simulink model "IEEE_IAS_H7_LoadCurrentRefVariation"  (Simulink 9.1)
settings: Solver=VariableStepAuto  StartTime=0.0  StopTime=0.2  RelTol=1e-3
libraries: powerlib x36, powerlib_extras x3, powerlib_meascontrol x3
settings Model: Creator=mohua  LastModifiedBy=mohua
settings DataIOCC: SaveFormat=Dataset
settings OptimizationCC: LifeSpan=auto
settings DebuggingCC: UnderspecifiedInitializationDetection=Simplified  MergeDetectMultiDrivingBlocksExec=error  SFUnexpectedBacktrackingDiag=error  SFNoUnconditionalDefaultTransitionDiag=error  SFExecutionAtInitializationDiag=warning
settings HardwareCC: ProdBitPerPointer=64  ProdBitPerSizeT=64  ProdBitPerPtrDiffT=64  ProdLargestAtomicFloat=Float  ProdIntDivRoundTo=Zero  ProdEndianess=LittleEndian  ProdWordSize=64  ProdHWDeviceType=Intel->x86-64 (Windows64)
settings ModelReferenceCC: PropagateSignalLabelsOutOfModel=on
settings CodeAppCC: StateflowObjectComments=off
settings GRTTargetCC: TargetLangStandard=C99 (ISO)  CombineOutputUpdateFcns=on  GRTInterface=off
settings ConfigComp: CovMetricSettings=dwe  CovHtmlReporting=off  CovSaveCumulativeToWorkspaceVar=off  CovSaveSingleToWorkspaceVar=off  CovExternalEMLEnable=on

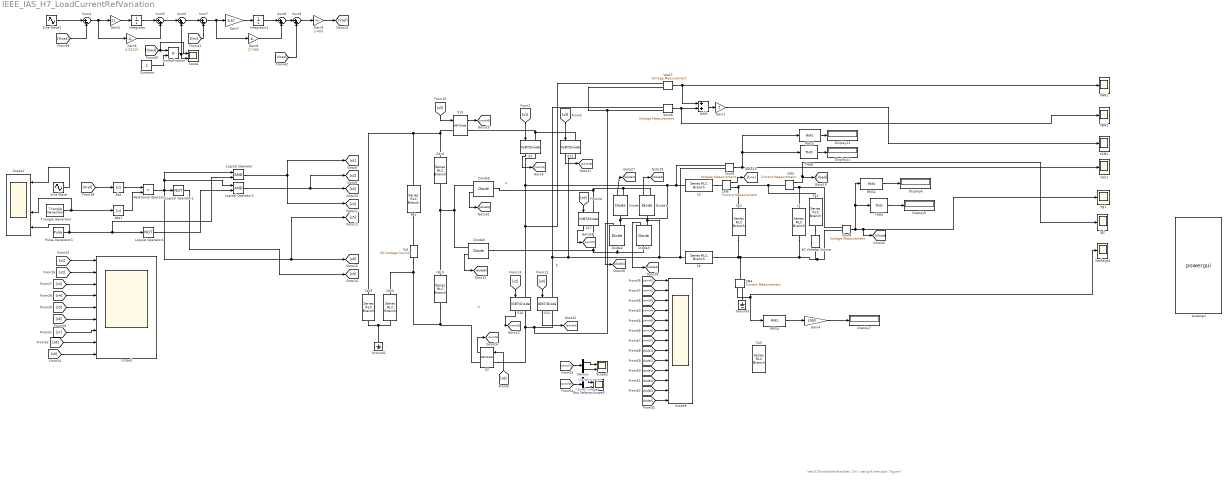
== system IEEE_IAS_H7_LoadCurrentRefVariation ==
  note: B
  note: A
  note: N
  note: set(0,'ShowHiddenHandles','On');
      | set(gcf,'menubar','figure')
  AC Voltage Source : powerlib/Electrical Sources/AC Voltage Source  Amplitude=311  Phase=0  Frequency=50  SampleTime=0  Measurements=None  BusType=swing  Pref=10e3  Qref=0  Qmin=-inf  Qmax=+inf
  Abs : Abs
  Abs1 : Abs
  Add1 : Sum
  Bus Selector : BusSelector  OutputSignals=Switch current,Switch voltage
  CM3 : powerlib/Measurements/Current Measurement  PhasorSimulation=off  OutputType=Complex  PSBequivalent=0
  CM4 : powerlib/Measurements/Current Measurement  PhasorSimulation=off  OutputType=Complex  PSBequivalent=0
  CM6 : powerlib/Measurements/Current Measurement  PhasorSimulation=off  OutputType=Complex  PSBequivalent=0
  Cdc3 : powerlib/Elements/Series RLC Branch  LConnTagsString=__new0  RConnTagsString=__new0  BranchType=C  Resistance=1  Inductance=3e-3  SetiL0=off  InitialCurrent=0  Capacitance=940e-6  Setx0=off  InitialVoltage=0  Measurements=None
  Cdc4 : powerlib/Elements/Series RLC Branch  LConnTagsString=__new0  RConnTagsString=__new0  BranchType=C  Resistance=1  Inductance=3e-3  SetiL0=off  InitialCurrent=0  Capacitance=940e-6  Setx0=off  InitialVoltage=0  Measurements=None
  Co1 : powerlib/Elements/Series RLC Branch  LConnTagsString=__new0  RConnTagsString=__new0  BranchType=C  Resistance=1  Inductance=3e-3  SetiL0=off  InitialCurrent=0  Capacitance=2.2e-6  Setx0=off  InitialVoltage=0  Measurements=None
  Co2 : powerlib/Elements/Series RLC Branch  LConnTagsString=__new0  RConnTagsString=__new0  BranchType=R  Resistance=0.001  Inductance=3e-3  SetiL0=off  InitialCurrent=0  Capacitance=2.2e-6  Setx0=off  InitialVoltage=0  Measurements=None
  Co5 : powerlib/Elements/Series RLC Branch  LConnTagsString=__new0  RConnTagsString=__new0  BranchType=R  Resistance=15  Inductance=3e-3  SetiL0=off  InitialCurrent=0  Capacitance=2.2e-6  Setx0=off  InitialVoltage=0  Measurements=None
  Constant : Constant  Value=2
  Cpv3 : powerlib/Elements/Series RLC Branch  LConnTagsString=__new0  RConnTagsString=__new0  BranchType=C  Resistance=1  Inductance=3e-3  SetiL0=off  InitialCurrent=0  Capacitance=75e-9  Setx0=off  InitialVoltage=0  Measurements=None
  Cpv4 : powerlib/Elements/Series RLC Branch  LConnTagsString=__new0  RConnTagsString=__new0  BranchType=C  Resistance=1  Inductance=3e-3  SetiL0=off  InitialCurrent=0  Capacitance=75e-9  Setx0=off  InitialVoltage=0  Measurements=None
  Demux : Demux  Outputs=2
  Diode{,1..3,8..9} (6 alike) : powerlib/Power Electronics/Diode  Ron=0.001  Lon=0  Vf=0.8  IC=0  UseSnubber=0  Rs=500  Cs=250e-9  Measurements=on
  Display{6..7,9,11..12} (5 alike) : Display
  Gain1 : Gain  Gain=.5
  Gain4 : Gain  Gain=1000
  Gain5 : Gain  Gain=21
  Gain6 : Gain  Gain=0.03115
  Gain7 : Gain  Gain=6.67
  Gain8 : Gain  Gain=27.066
  Gain9 : Gain  Gain=1/400
  Ground2 : powerlib/Elements/Ground  LConnTagsString=a
  Ground3 : powerlib/Elements/Ground  LConnTagsString=a
  Ig2 : Scope
  Ileakage1 : Scope
  Integrator : Integrator
  Integrator1 : Integrator
  L1 : powerlib/Elements/Series RLC Branch  LConnTagsString=__new0  RConnTagsString=__new0  BranchType=RL  Resistance=2000  Inductance=100  SetiL0=off  InitialCurrent=0  Capacitance=1e-6  Setx0=off  InitialVoltage=0  Measurements=None
  L3 : powerlib/Elements/Series RLC Branch  LConnTagsString=__new0  RConnTagsString=__new0  BranchType=L  Resistance=1  Inductance=3e-3  SetiL0=off  InitialCurrent=0  Capacitance=1e-6  Setx0=off  InitialVoltage=0  Measurements=None
  L4 : powerlib/Elements/Series RLC Branch  LConnTagsString=__new0  RConnTagsString=__new0  BranchType=L  Resistance=1  Inductance=3e-3  SetiL0=off  InitialCurrent=0  Capacitance=1e-6  Setx0=off  InitialVoltage=0  Measurements=None
  Logical Operator : Logic  AllPortsSameDT=off  OutDataTypeStr=boolean
  Logical Operator1 : Logic  Operator=NOT  AllPortsSameDT=off  OutDataTypeStr=boolean
  Logical Operator2 : Logic  AllPortsSameDT=off  OutDataTypeStr=boolean
  Logical Operator4 : Logic  Operator=NOT  AllPortsSameDT=off  OutDataTypeStr=boolean
  Pulse Generator1 : DiscretePulseGenerator  PulseType=Time based  Period=.02  PulseWidth=50
  RMS2 : powerlib_extras/Measurements/RMS  f1=50
  RMS4 : powerlib_extras/Measurements/RMS  f1=50
  RMS5 : powerlib_extras/Measurements/RMS  f1=50
  Relational Operator : RelationalOperator  Operator=>  OutDataTypeStr=boolean  RndMeth=Nearest
  Rs1 : powerlib/Elements/Series RLC Branch  LConnTagsString=__new0  RConnTagsString=__new0  BranchType=R  Resistance=1  Inductance=3e-3  SetiL0=off  InitialCurrent=0  Capacitance=1e-6  Setx0=off  InitialVoltage=0  Measurements=None
  S{2..3,10..13,17} (7 alike) : powerlib/Power Electronics/IGBT//Diode  Ron=1e-3  Rs=1e5  Cs=inf  Measurements=on
  Scope : Scope  NumInputPorts=2
  Scope1 : Scope  NumInputPorts=4
  Scope2 : Scope  NumInputPorts=2
  Scope3 : Scope  NumInputPorts=2
  Scope8 : Scope  NumInputPorts=13
  Sine Wave : Sin  Frequency=2*pi*50  SampleTime=0
  Sine Wave2 : Sin  Amplitude=350  Frequency=2*pi*50  SampleTime=0
  Sum4 : Sum  Inputs=|+-
  Sum{5..6,8..9} (4 alike) : Sum  Inputs=|++
  Sum7 : Sum  Inputs=|+-
  THD5 : powerlib_meascontrol/Measurements/THD  Freq=50  Ts=0
  THD6 : powerlib_meascontrol/Measurements/THD  Freq=60  Ts=0
  Triangle Generator : powerlib_meascontrol/Pulse & Signal Generators/Triangle Generator  Freq=20e3  Phase=90  Ts=0
  VAN1 : Scope
  VBN1 : Scope
  VCM1 : Scope
  Vab1 : Scope
  Vg1 : Scope
  Vout{6..9} (4 alike) : powerlib/Measurements/Voltage Measurement  PhasorSimulation=off  OutputType=Complex  PSBequivalent=0
  Vs1 : powerlib/Electrical Sources/DC Voltage Source  Amplitude=400  Measurements=None
  multiplication : Product  SaturateOnIntegerOverflow=on  RndMeth=Zero
  powergui : powerlib/powergui  Priority=1  SimulationMode=Continuous  SampleTime=50e-6  frequency=60  Iterations=50  frequencyindice=0  Pbase=100e6  ErrMax=1e-4  UnitsV=kV  UnitsW=MW  buscounter=0  FunctionMessages=off  echomessages=off  EnableUseOfTLC=off  CurrentSourceSwitches=off  DisableSnubberDevices=off  DisableRonSwitches=off  DisableVfSwitches=off  DisplayEquations=off  SolverType=Tustin/Backward Euler (TBE)  Interpol=off  ExternalGateDelay=off  methode=off  Ts=100  x0status=blocks  SPID=on  SwTol=0  HookPort=off  RestoreLinks=warning  ResistiveCurrentMeasurement=off  Frange=[0:2:500]  Ylog=off  Xlog=on  ShowGrid=off  save=off  variable=ZData  structure=voltage  ZoomFFT=off  StartTime=0.5  cycles=10  DisplayStyle=2  fundamental=50  FreqAxis=off  MaxFrequency=1000  frequencyindicesteady=1  RmsSteady=1  display=off
  scope1 : Scope  NumInputPorts=9
  wires:
  Sum4/1 -> Gain6/1, Gain5/1
  THD6/1 -> Display11/1
  Bus Selector/2 -> Scope3/2  "<Switch voltage>"
  [swirch5] -> Scope8/5
  [diode3] -> Scope8/10
  S17/1 -> [swirch7]
  Gain1/1 -> VCM1/1
  [diode5] -> Scope8/12
  [s4] -> scope1/4
  Diode/1 -> [diode1]
  S3/1 -> [swirch1]
  [s7] -> scope1/7
  Demux/1 -> Scope2/1
  [diode4] -> Scope8/11
  S10/1 -> [swirch2]
  [diode6] -> Scope8/13
  RMS5/1 -> Display12/1
  Vout9/1 -> RMS5/1, THD6/1, Vab1/1
  Diode8/1 -> [diode6]
  [diode2] -> Scope8/9
  [s5] -> S13/1
  [swirch2] -> Bus Selector/1
  [swirch2] -> Scope8/2
  S12/1 -> [swirch4]
  [Iload] -> multiplication/1, Scope/1
  [swirch7] -> Scope8/7
  Relational Operator/1 -> Logical Operator2/1, Logical Operator/1, [s5], [s8], Logical Operator1/1
  [swirch1] -> Scope8/1
  [swirch3] -> Scope8/3
  [swirch4] -> Scope8/4
  Diode9/1 -> [diode5]
  S13/1 -> [swirch5]
  Gain5/1 -> Integrator/1
  RMS2/1 -> Display6/1
  Sum9/1 -> Gain9/1
  [diode1] -> Scope8/8
  Diode2/1 -> [diode2]
  [Vload] -> Sum9/2
  Diode3/1 -> [diode4]
  Abs1/1 -> Relational Operator/2
  Gain6/1 -> Sum5/2
  Gain4/1 -> Display7/1
  Sum5/1 -> Sum6/1
  Integrator/1 -> Sum5/1
  [Vload] -> Sum4/2
  Sum7/1 -> Gain8/1, Gain7/1
  Sum8/1 -> Sum9/1
  Gain9/1 -> [Vref]
  [swirch6] -> Scope8/6
  [s9] -> S17/1
  Gain8/1 -> Sum8/2
  [s2] -> scope1/2
  Integrator1/1 -> Sum8/1
  Gain7/1 -> Integrator1/1
  S2/1 -> [swirch6]
  [Vref] -> Abs/1
  [s9] -> scope1/9
  Logical Operator/1 -> [s1], [s4]
  CM4/1 -> RMS4/1, Ileakage1/1
  Sum6/1 -> Sum7/1
  Triangle Generator/1 -> Scope1/3, Abs1/1
  [s8] -> S2/1
  [s8] -> scope1/8
  [s1] -> scope1/1
  Abs/1 -> Relational Operator/1
  Sine Wave/1 -> Scope1/1
  Vout8/1 -> VBN1/1, Add1/2
  [s4] -> S12/1
  [s6] -> scope1/6
  Add1/1 -> Gain1/1
  Logical Operator4/1 -> Logical Operator2/2
  Vout7/1 -> Add1/1, VAN1/1
  [s5] -> scope1/5
  Diode1/1 -> [diode3]
  [s2] -> S10/1
  CM3/1 -> [Iload], Ig2/1
  RMS4/1 -> Gain4/1
  [s3] -> S11/1
  [Iinv] -> Sum7/2
  [s1] -> S3/1
  Bus Selector/1 -> Scope3/1  "<Switch current>"
  Pulse Generator1/1 -> Scope1/4, Logical Operator/2, Logical Operator4/1
  Vout6/1 -> THD5/1, RMS2/1, [Vload], Vg1/1
  S11/1 -> [swirch3]
  THD5/1 -> Display9/1
  [swirch1] -> Demux/1
  Sine Wave2/1 -> Sum4/1
  CM6/1 -> [Iinv]
  Logical Operator2/1 -> [s3], [s2]
  [s3] -> scope1/3
  Logical Operator1/1 -> [s9]
  Demux/2 -> Scope2/2
  multiplication/1 -> Scope/2, Sum6/2
  Constant/1 -> multiplication/2
  connections:
  S10/LConn1 -- S3/RConn1 -- Vout9/LConn1 -- L3/LConn1 -- Diode/LConn1 -- Diode2/RConn1 -- Vout7/LConn1
  Rs1/RConn1 -- S13/LConn1 -- Cdc4/LConn1 -- Cpv3/LConn1
  Cdc3/RConn1 -- S2/RConn1 -- Cpv4/LConn1 -- Vs1/LConn1
  Diode1/LConn1 -- Diode3/RConn1 -- L4/LConn1 -- Vout9/LConn2 -- S11/RConn1 -- S12/LConn1 -- Vout8/LConn1
  L4/RConn1 -- AC Voltage Source/LConn1 -- Vout6/LConn2 -- L1/RConn1 -- CM4/LConn1 -- Co1/RConn1
  Diode8/LConn1 -- S17/RConn1 -- Diode3/LConn1 -- Diode2/LConn1
  Cpv3/RConn1 -- Ground2/LConn1 -- Cpv4/RConn1
  Cdc3/LConn1 -- Diode9/RConn1 -- Diode8/RConn1 -- Cdc4/RConn1
  Diode/RConn1 -- S17/LConn1 -- Diode9/LConn1 -- Diode1/RConn1
  Vout6/LConn1 -- L1/LConn1 -- CM3/RConn1
  CM6/RConn1 -- Co1/LConn1 -- Co2/LConn1 -- CM3/LConn1
  Vout7/LConn2 -- Vout8/LConn2 -- S12/RConn1 -- S2/LConn1 -- S10/RConn1
  S11/LConn1 -- S3/LConn1 -- S13/RConn1
  L3/RConn1 -- CM6/LConn1
  Rs1/LConn1 -- Vs1/RConn1
  Ground3/LConn1 -- CM4/RConn1
  Co2/RConn1 -- AC Voltage Source/RConn1
